simulink model "Controllo_modello_OL"  (R2024a)
settings: Solver=FixedStepAuto  StartTime=tempo(1)  StopTime=tempo(end)  FixedStep=1e-3  RelTol=1e-3
undefined symbols (not defined in the file): alpha_0, alpha_dot_0, cc, cm, dinamica_alpha, g, L, mc, mm, xc_0, xc_dot_0
libraries: simulink x2
settings Model: Creator=smila  LastModifiedBy=smila
settings OptimizationCC: BlockReduction=off  DefaultParameterBehavior=Inlined  BufferReuse=off

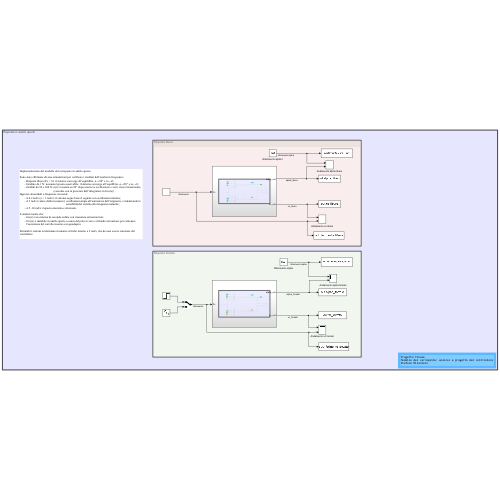
[thumbnail: Simulink's stored preview of the top-level diagram]
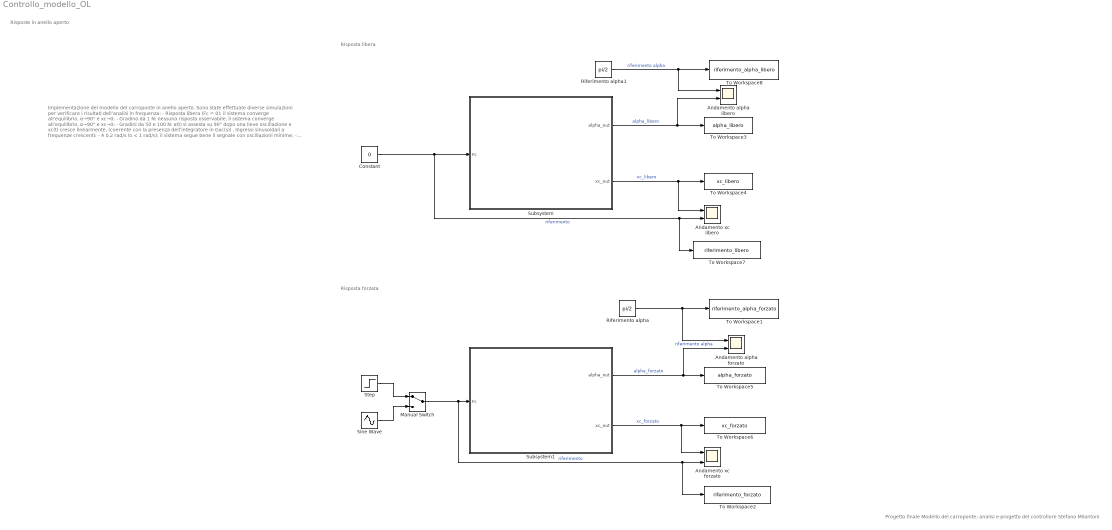
== system Controllo_modello_OL ==
  note: Risposta libera
  note: Implementazione del modello del carroponte in anello aperto.
      | Sono state effettuate diverse simulazioni per verificare i risultati dell’analisi in frequenza:
      | - Risposta libera (Fc = 0): il sistema converge all’equilibrio, α→90° e xc→0;
      | - Gradino da 1 N: nessuna risposta osservabile, il sistema converge all’equilibrio, α→90° e xc→0;
      | - Gradini da 50 e 100 N: α(t) si assesta su 90° dopo una lieve oscillazione e xc(t) cresce linearmente, (coerente con la presenza dell’integratore in Gxc(s)) .
      | Ingressi sinusoidali a frequenze crescenti:
      | - A 0.2 rad/s (o < 1 rad/s): il sistema segue bene il segnale con oscillazioni minime;
      | - A 2 rad/s (valore della risonanza): oscillazioni ampie all’aumentare dell’ampiezza, evidenziando la sensibilità del sistema alla frequenza naturale;
      | - A 5–10 rad/s: risposta smorzata e attenuata.
      | L’analisi mostra che:
      | - Gα(s) è un sistema di secondo ordine con risonanza sottosmorzata;
      | - Gxc(s) è instabile in anello aperto a causa del polo in zero e richiede retroazione per contenere l’escursione del carrello inseme a un guadagno;
      |
      | Entrambi i sistemi evidenziano risonanze critiche intorno a 2 rad/s, che devono essere smorzate dal controllore.
  note: Risposte in anello aperto
  note: Progetto finale
      | Modello del carroponte: analisi e progetto del controllore
      | Stefano Milantoni
  note: Risposta forzata
  Andamento alpha forzato : Scope  NumInputPorts=2
  Andamento alpha libero : Scope  NumInputPorts=2
  Andamento xc forzato : Scope  NumInputPorts=2
  Andamento xc libero : Scope  NumInputPorts=2
  Constant : Constant  Value=0
  Manual Switch : ManualSwitch
  Riferimento alpha : Constant  Value=pi/2
  Riferimento alpha1 : Constant  Value=pi/2
  Sine Wave : Sin  Amplitude=1e3  Frequency=2  SampleTime=0
  Step : Step  Time=15  SampleTime=0
  Subsystem : Subsystem
  Subsystem1 : Subsystem
  To Workspace1 : ToWorkspace  VariableName=riferimento_alpha_forzato  SaveFormat=Structure With Time  SampleTime=-1
  To Workspace2 : ToWorkspace  VariableName=riferimento_forzato  SaveFormat=Structure With Time  SampleTime=-1
  To Workspace3 : ToWorkspace  VariableName=alpha_libero  SaveFormat=Structure With Time  SampleTime=-1
  To Workspace4 : ToWorkspace  VariableName=xc_libero  SaveFormat=Structure With Time  SampleTime=-1
  To Workspace5 : ToWorkspace  VariableName=alpha_forzato  SaveFormat=Structure With Time  SampleTime=-1
  To Workspace6 : ToWorkspace  VariableName=xc_forzato  SaveFormat=Structure With Time  SampleTime=-1
  To Workspace7 : ToWorkspace  VariableName=riferimento_libero  SaveFormat=Structure With Time  SampleTime=-1
  To Workspace8 : ToWorkspace  VariableName=riferimento_alpha_libero  SaveFormat=Structure With Time  SampleTime=-1
  wires:
  Subsystem/2(xc_out) -> Andamento xc libero/1, To Workspace4/1  "xc_libero"
  Subsystem1/1(alpha_out) -> Andamento alpha forzato/2, To Workspace5/1  "alpha_forzato"
  Subsystem1/2(xc_out) -> Andamento xc forzato/1, To Workspace6/1  "xc_forzato"
  Subsystem/1(alpha_out) -> To Workspace3/1, Andamento alpha libero/2  "alpha_libero"
  Constant/1 -> To Workspace7/1, Andamento xc libero/2, Subsystem/1(Fc)  "riferimento"
  Manual Switch/1 -> To Workspace2/1, Andamento xc forzato/2, Subsystem1/1(Fc)  "riferimento"
  Step/1 -> Manual Switch/1
  Sine Wave/1 -> Manual Switch/2
  Riferimento alpha/1 -> To Workspace1/1, Andamento alpha forzato/1  "riferimento alpha"
  Riferimento alpha1/1 -> Andamento alpha libero/1, To Workspace8/1  "riferimento alpha"

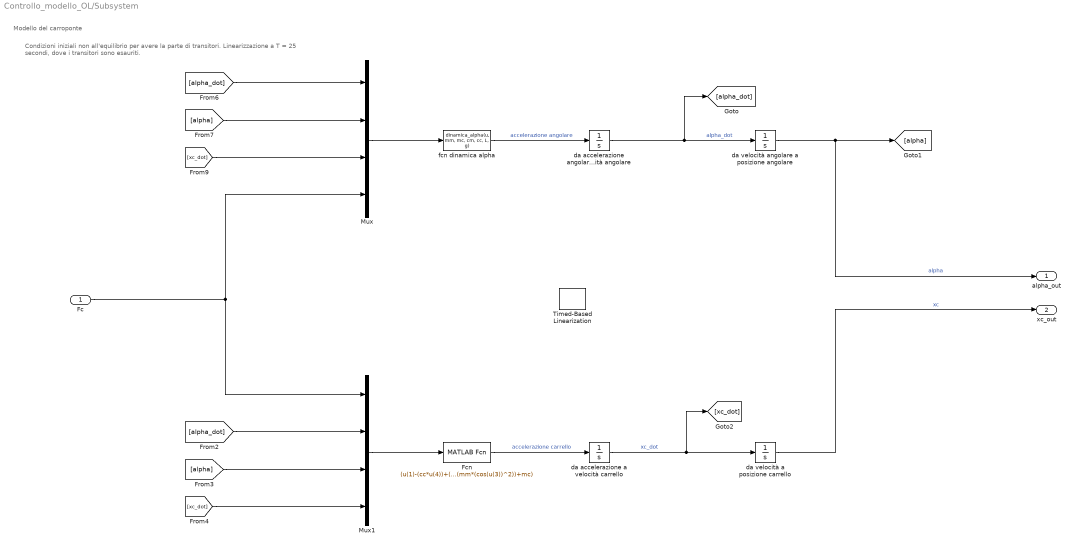
== system Controllo_modello_OL/Subsystem ==
  note: Condizioni iniziali non all'equilibrio per avere la parte di transitori.
      | Linearizzazione a T = 25 secondi, dove i transitori sono esauriti.
  note: Modello del carroponte
  Fc : Inport
  Fcn : MATLABFcn  MATLABFcn=(u(1)-(cc*u(4))+(mm*g*sin(u(3))*cos(u(3)))-(cm*u(4)*(cos(u(3))^2))+(mm*L*cos(u(3))*(u(2)^2)))/((mm*(cos(u(3))^2))+mc)
  Mux : Mux
  Mux1 : Mux
  Timed-Based Linearization : simulink/Model-Wide Utilities/Timed-Based Linearization  LinearizationTime=25  SampleTime=0
  da accelerazione a velocità carrello : Integrator  InitialCondition=xc_dot_0
  da accelerazione angolare a velocità angolare : Integrator  InitialCondition=alpha_dot_0
  da velocità a posizione carrello : Integrator  InitialCondition=xc_0
  da velocità angolare a posizione angolare : Integrator  InitialCondition=alpha_0
  fcn dinamica alpha : MATLABFcn  MATLABFcn=dinamica_alpha(u, mm, mc, cm, cc, L, g)
  alpha_out : Outport
  xc_out : Outport  Port=2
  wires:
  fcn dinamica alpha/1 -> da accelerazione angolare a velocità angolare/1  "accelerazione angolare"
  da accelerazione a velocità carrello/1 -> da velocità a posizione carrello/1, [xc_dot]  "xc_dot"
  da accelerazione angolare a velocità angolare/1 -> da velocità angolare a posizione angolare/1, [alpha_dot]  "alpha_dot"
  Fcn/1 -> da accelerazione a velocità carrello/1  "accelerazione carrello"
  da velocità angolare a posizione angolare/1 -> alpha_out/1, [alpha]  "alpha"
  Fc/1 -> Mux/4, Mux1/1
  da velocità a posizione carrello/1 -> xc_out/1  "xc"
  [alpha_dot] -> Mux1/2
  [alpha_dot] -> Mux/1
  Mux/1 -> fcn dinamica alpha/1
  Mux1/1 -> Fcn/1
  [xc_dot] -> Mux/3
  [alpha] -> Mux/2
  [alpha] -> Mux1/3
  [xc_dot] -> Mux1/4

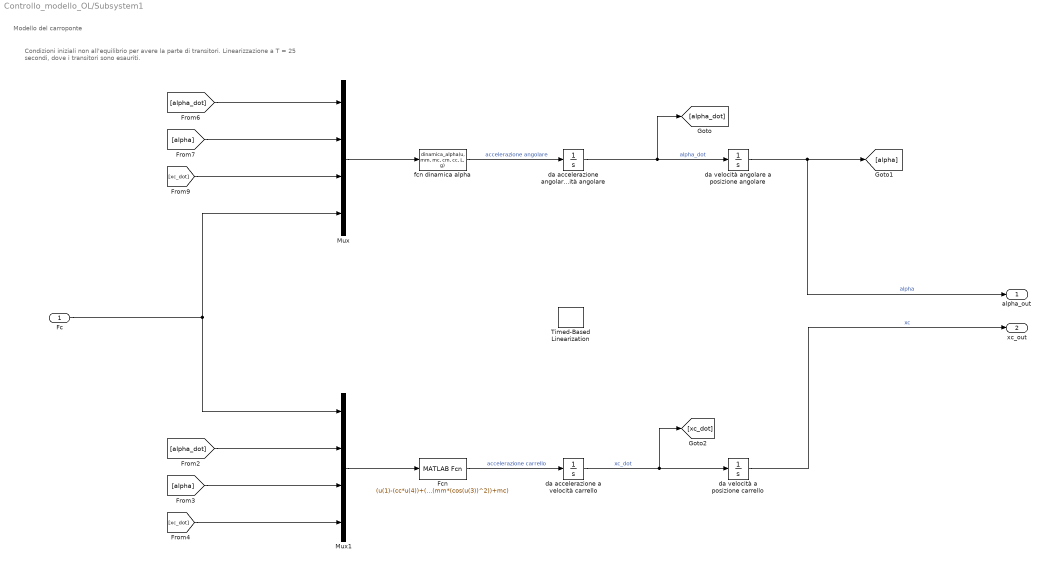
== system Controllo_modello_OL/Subsystem1 ==
  note: Condizioni iniziali non all'equilibrio per avere la parte di transitori.
      | Linearizzazione a T = 25 secondi, dove i transitori sono esauriti.
  note: Modello del carroponte
  Fc : Inport
  Fcn : MATLABFcn  MATLABFcn=(u(1)-(cc*u(4))+(mm*g*sin(u(3))*cos(u(3)))-(cm*u(4)*(cos(u(3))^2))+(mm*L*cos(u(3))*(u(2)^2)))/((mm*(cos(u(3))^2))+mc)
  Mux : Mux
  Mux1 : Mux
  Timed-Based Linearization : simulink/Model-Wide Utilities/Timed-Based Linearization  LinearizationTime=25  SampleTime=0
  da accelerazione a velocità carrello : Integrator  InitialCondition=xc_dot_0
  da accelerazione angolare a velocità angolare : Integrator  InitialCondition=alpha_dot_0
  da velocità a posizione carrello : Integrator  InitialCondition=xc_0
  da velocità angolare a posizione angolare : Integrator  InitialCondition=alpha_0
  fcn dinamica alpha : MATLABFcn  MATLABFcn=dinamica_alpha(u, mm, mc, cm, cc, L, g)
  alpha_out : Outport
  xc_out : Outport  Port=2
  wires:
  fcn dinamica alpha/1 -> da accelerazione angolare a velocità angolare/1  "accelerazione angolare"
  da accelerazione a velocità carrello/1 -> da velocità a posizione carrello/1, [xc_dot]  "xc_dot"
  da accelerazione angolare a velocità angolare/1 -> da velocità angolare a posizione angolare/1, [alpha_dot]  "alpha_dot"
  Fcn/1 -> da accelerazione a velocità carrello/1  "accelerazione carrello"
  da velocità angolare a posizione angolare/1 -> alpha_out/1, [alpha]  "alpha"
  Fc/1 -> Mux/4, Mux1/1
  da velocità a posizione carrello/1 -> xc_out/1  "xc"
  [alpha_dot] -> Mux1/2
  [alpha_dot] -> Mux/1
  Mux/1 -> fcn dinamica alpha/1
  Mux1/1 -> Fcn/1
  [xc_dot] -> Mux/3
  [alpha] -> Mux/2
  [alpha] -> Mux1/3
  [xc_dot] -> Mux1/4
